simulink model "nomoto_model_nonlinear"  (R2015a)
settings: Solver=ode45  StartTime=0.0  StopTime=tstop  RelTol=1e-3
values from neighbouring files (symbols this model uses):
  c_ss = lsqcurvefit(p, c_0, r_tests, d_c_tests)    [run.m]
  d_c = 1 * (pi/180)    (= 0.0174532925199)    [run.m]
  K = c_f(1) / d_c    [run.m]
  T = 1 / c_f(2)    [run.m]
  tsamp = 10    [run.m]
settings Model: Creator=patrickf  LastModifiedBy=patrickf

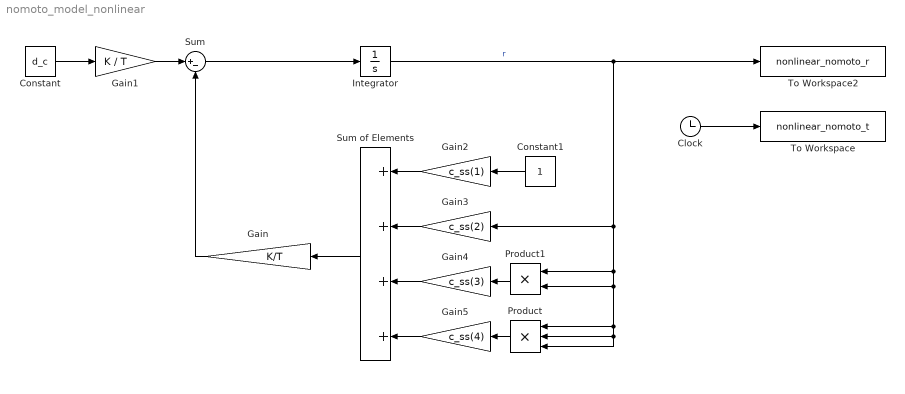
== system nomoto_model_nonlinear ==
  Clock : Clock
  Constant : Constant  Value=d_c
  Constant1 : Constant
  Gain : Gain  Gain=K/T
  Gain1 : Gain  Gain=K / T
  Gain2 : Gain  Gain=c_ss(1)
  Gain3 : Gain  Gain=c_ss(2)
  Gain4 : Gain  Gain=c_ss(3)
  Gain5 : Gain  Gain=c_ss(4)
  Integrator : Integrator
  Product : Product  Inputs=3
  Product1 : Product
  Sum : Sum  Inputs=|+-
  Sum of Elements : Sum  Inputs=4
  To Workspace : ToWorkspace  VariableName=nonlinear_nomoto_t  SampleTime=tsamp
  To Workspace2 : ToWorkspace  VariableName=nonlinear_nomoto_r  SampleTime=tsamp
  wires:
  Sum/1 -> Integrator/1
  Gain/1 -> Sum/2
  Constant/1 -> Gain1/1
  Gain1/1 -> Sum/1
  Clock/1 -> To Workspace/1
  Sum of Elements/1 -> Gain/1
  Gain3/1 -> Sum of Elements/2
  Gain4/1 -> Sum of Elements/3
  Gain5/1 -> Sum of Elements/4
  Gain2/1 -> Sum of Elements/1
  Integrator/1 -> To Workspace2/1, Gain3/1, Product/3, Product/2, Product/1, Product1/2, Product1/1  "r"
  Constant1/1 -> Gain2/1
  Product1/1 -> Gain4/1
  Product/1 -> Gain5/1
